simulink model "Appl_HeatAdj_CtrlModel"  (R2018b)
settings: configuration reference "CodeConfig_10_ms" (kept outside this file)
undefined symbols (not defined in the file): CAL_LEVEL3_TIMEOUT, CAL_SW_20min_TIMEOUT, D_1stLevel_36, D_2ndLevel_39, D_3rdLevel_45, D_3rdLevel_48, D_DRVHEAT_PID_D, D_DRVHEAT_PID_I, D_DRVHEAT_PID_P, D_HEAT_HEAT_DEF, D_SwsLevel_Temp, FALSE, TRUE
libraries: DareLib x111, simulink x1
(part 6 of 6)

== stateflow chart Appl_HeatAdj_CtrlModel/LogicCtrl/LocalAdjustCtrl/OutputDeal/TempFunction2/TempFunction ==
  state Ts = D_HAL_GET_CUR_MS_TS [function]
  state OutTs = TimeDiffTs(lastTs,Ts) [function]
  state TempLvl
    (default) -> (junction 39)
    TempLvl -> (junction 39)
    (junction 39) -> (junction 41) [order 1] : /* P20方向盘加热等级 */
        | [enProjectType.EN_PROJECT_P20 == ProjectType ...
        | && TRUE == ThirdHeat]
    (junction 39) -> (junction 6) [order 2]
    (junction 41) -> (junction 43) : {AimTemp = D_SwsLevel_Temp;
        | TimeCnt = D_HAL_GET_CUR_MS_TS();}
    (junction 6) -> (junction 8) [order 1] : /* 等级1 */
        | [enHeatLvlSts.EN_HEAT_LVL_1 == AimLevel]
    (junction 6) -> (junction 10) [order 2]
    (junction 8) -> (junction 24) : {AimTemp = D_1stLevel_36;
        | TimeCnt = D_HAL_GET_CUR_MS_TS();}
    (junction 10) -> (junction 12) [order 1] : /* 等级2 */
        | [enHeatLvlSts.EN_HEAT_LVL_2 == AimLevel]
    (junction 10) -> (junction 14) [order 2]
    (junction 12) -> (junction 22) : {AimTemp = D_2ndLevel_39;
        | TimeCnt = D_HAL_GET_CUR_MS_TS();}
    (junction 14) -> (junction 16) [order 1] : /* 等级3 */
        | [enHeatLvlSts.EN_HEAT_LVL_3 == AimLevel]
    (junction 14) -> (junction 18) [order 2] : {AimTemp = 0;
        | TimeCnt = D_HAL_GET_CUR_MS_TS();}
    (junction 16) -> (junction 49)
    (junction 49) -> (junction 50) [order 1] : /* 小于13min 且为P20 且本次未降至 45度(防止32bit计数超时重新小于13min) */
        | [enProjectType.EN_PROJECT_P20 == ProjectType ...
        | && TimeDiffTs(TimeCnt,D_HAL_GET_CUR_MS_TS()) <= CAL_LEVEL3_TIMEOUT ...
        | && AimTemp != D_3rdLevel_45]
    (junction 49) -> (junction 20) [order 2] : {AimTemp = D_3rdLevel_45;}
    (junction 50) -> (junction 52) : {AimTemp = D_3rdLevel_48;}
    (junction 20) -> (junction 18)
    (junction 52) -> (junction 20)
    (junction 22) -> (junction 52)
    (junction 24) -> (junction 22)
    (junction 43) -> (junction 24)
    (junction 18) -> (junction 29)
  (default) -> TempLvl
  data: Ts function_output; lastTs function_input; Ts function_input; OutTs function_output; AimTemp output uint16; D_1stLevel_36 parameter; D_2ndLevel_39 parameter; AimLevel input Enum: enHeatLvlSts; ProjectType input uint8; ThirdHeat input uint8; D_SwsLevel_Temp parameter; TRUE parameter; TimeCnt local uint32; CAL_LEVEL3_TIMEOUT parameter; D_3rdLevel_45 parameter; D_3rdLevel_48 parameter

== stateflow chart Appl_HeatAdj_CtrlModel/LogicCtrl/LocalAdjustCtrl/OutputDeal/TempFunction2/TempFunction/TimeDiffTs/Chart ==
  (default) -> (junction 3)
  (junction 3) -> (junction 5)
  (junction 5) -> (junction 7) [order 1] : /* 入参比当前大 */
      | [lastTs > Ts]
  (junction 5) -> (junction 13) [order 2] : {OutTs = Ts - lastTs;}
  (junction 7) -> (junction 11) : {OutTs = 0xFFFFFFFF - lastTs + Ts +1;}
  (junction 11) -> (junction 13)
  (junction 13) -> (junction 17)
  data: lastTs input uint32; Ts input uint32; OutTs output uint32
